simulink model "prob1_part1_link"  (R2016a)
settings: Solver=VariableStepAuto  StartTime=0.0  StopTime=10.0  RelTol=1e-3
settings Model: Creator=Brad  LastModifiedBy=Brad

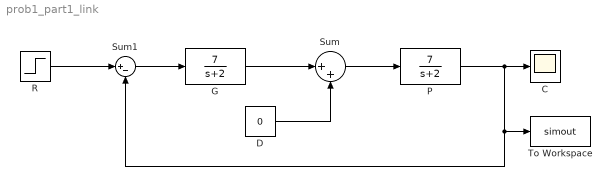
== system prob1_part1_link ==
  C : Scope
  D : Constant  Value=0
  G : TransferFcn  Numerator=[7]  Denominator=[1 2]
  P : TransferFcn  Numerator=[7]  Denominator=[1 2]
  R : Step  After=3  SampleTime=0
  Sum : Sum  Inputs=|++
  Sum1 : Sum  Inputs=|+-
  To Workspace : ToWorkspace  VariableName=simout  SaveFormat=Timeseries  SampleTime=-1
  wires:
  Sum/1 -> P/1
  D/1 -> Sum/2
  G/1 -> Sum/1
  Sum1/1 -> G/1
  P/1 -> C/1, To Workspace/1, Sum1/2
  R/1 -> Sum1/1
